simulink model "MSD_model"  (R2022b)
settings: Solver=VariableStepAuto  StartTime=0.0  StopTime=10.0  MaxStep=0.01  RelTol=1e-3
undefined symbols (not defined in the file or in its folder): b, k, m, x0
settings Model: Creator=Brigosha_Guest  LastModifiedBy=Brigosha_Guest

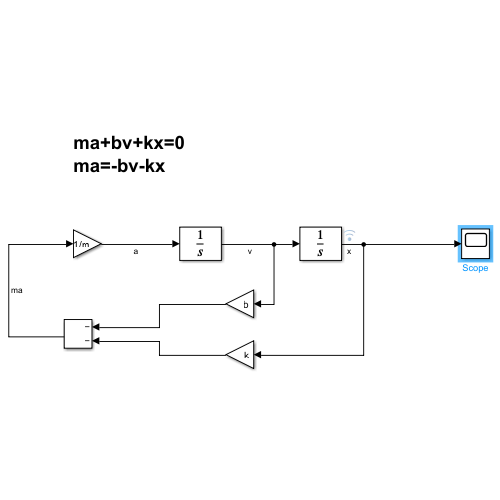
[thumbnail: Simulink's stored preview of the top-level diagram]
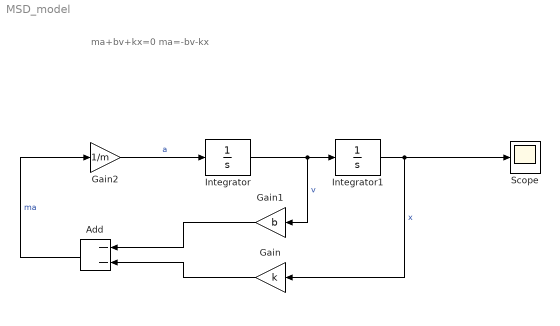
== system MSD_model ==
  note: ma+bv+kx=0
      | ma=-bv-kx
  Add : Sum  Inputs=--
  Gain : Gain  Gain=k
  Gain1 : Gain  Gain=b
  Gain2 : Gain  Gain=1/m
  Integrator : Integrator
  Integrator1 : Integrator  InitialCondition=x0
  Scope : Scope
  wires:
  Gain2/1 -> Integrator/1  "a"
  Integrator/1 -> Gain1/1, Integrator1/1  "v"
  Integrator1/1 -> Gain/1, Scope/1  "x"
  Gain1/1 -> Add/1
  Gain/1 -> Add/2
  Add/1 -> Gain2/1  "ma"
